simulink model "COPIA03052018"  (R2016a)
settings: Solver=ode3  StartTime=0.0  StopTime=inf  FixedStep=h  RelTol=1e-3
undefined symbols (not defined in the file): h, National_Instruments, PCI
libraries: sldrtlib x4, fuzblock x1
settings Model: SimulationMode=external  Creator=Jovani  LastModifiedBy=MCAC-UAEH
settings DataIOCC: LimitDataPoints=on  SaveFormat=Array
settings DebuggingCC: UnderspecifiedInitializationDetection=Classic  MergeDetectMultiDrivingBlocksExec=none  SolverPrmCheckMsg=warning  StateNameClashWarn=warning
settings HardwareCC: ProdBitPerLong=64  ProdLargestAtomicFloat=None  ProdHWDeviceType=Intel->x86-64  TargetBitPerLong=64  TargetBitPerPointer=64  TargetIntDivRoundTo=Zero  TargetEndianess=LittleEndian  TargetWordSize=64  TargetHWDeviceType=Intel->x86-64
settings ModelReferenceCC: PropagateSignalLabelsOutOfModel=off
settings RTWCC: SystemTargetFile=sldrt.tlc  TemplateMakefile=sldrt.tmf  Description=Simulink Desktop Real-Time  RTWCompilerOptimization=on
settings CodeAppCC: MaxIdLength=95
settings SimulinkDesktopRealTimeCC: TargetPreCompLibLocation=C:\Program Files\MATLAB\R2016a\toolbox\sldrt\lib\win64  TargetLangStandard=C89/C90 (ANSI)  SupportVariableSizeSignals=off
settings ConfigComp: CovModelRefEnable=Off

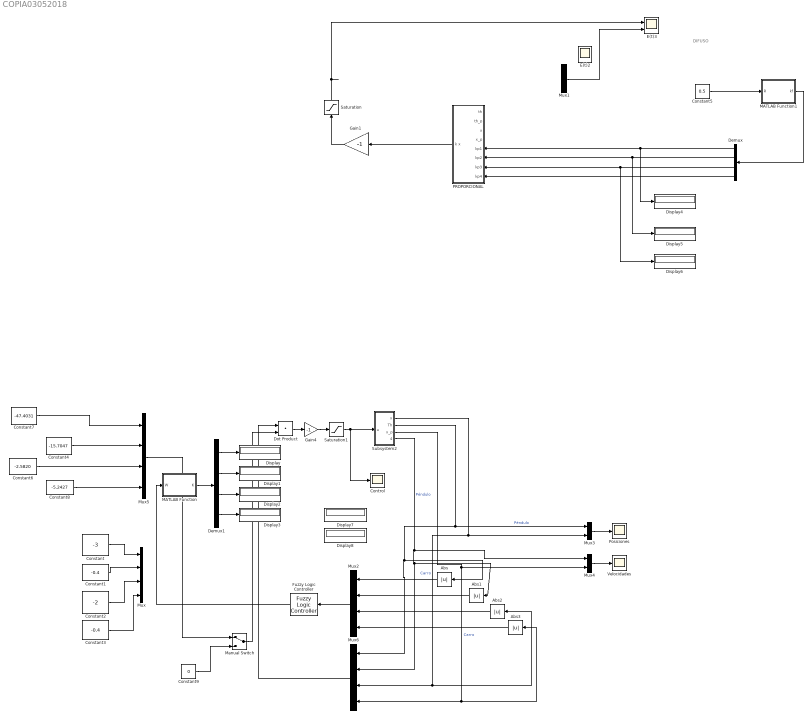
== system COPIA03052018 ==
  note: DIFUSO
  Abs{,1..3} (4 alike) : Abs
  Constant : Constant  Value=-3
  Constant1 : Constant  Value=-0.4
  Constant2 : Constant  Value=-2
  Constant3 : Constant  Value=-0.4
  Constant4 : Constant  Value=-15.7047
  Constant5 : Constant  Value=0.5
  Constant6 : Constant  Value=-2.5820
  Constant7 : Constant  Value=-47.4031
  Constant8 : Constant  Value=-5.2427
  Constant9 : Constant  Value=0
  "Control " : Scope
  Demux : Demux
  Demux1 : Demux
  Display{,1..8} (9 alike) : Display
  Dot Product : DotProduct  InputSameDT=on  OutDataTypeStr=Inherit: Inherit via internal rule
  E(t)2 : Scope  NumInputPorts=4
  E(t)3 : Scope  NumInputPorts=2
  Fuzzy Logic Controller : fuzblock/Fuzzy Logic  Controller  fis=P_T
  Gain1 : Gain  Gain=-1
  Gain4 : Gain  Gain=-1
  MATLAB Function : MATLAB Function  TreatAsAtomicUnit=on
  MATLAB Function1 : MATLAB Function  TreatAsAtomicUnit=on
  Manual Switch : ManualSwitch
  Mux{,1..2,5..6} (5 alike) : Mux
  Mux3 : Mux  Inputs=2
  Mux4 : Mux  Inputs=2
  PROPORCIONAL : Subsystem
  Posiciones : Scope
  Saturation : Saturate  UpperLimit=7.5  LowerLimit=-7.5
  Saturation1 : Saturate  UpperLimit=7.5  LowerLimit=-7.5
  Subsystem2 : Subsystem
  Velocidades : Scope
  wires:
  Gain1/1 -> Saturation/1
  ? -> PROPORCIONAL/2(th_p), Mux1/4, E(t)2/3
  ? -> E(t)2/4, Mux1/3, PROPORCIONAL/4(x_p)
  ? -> E(t)2/2, Mux1/2, PROPORCIONAL/1(th)
  ? -> E(t)2/1, Mux1/1, PROPORCIONAL/3(x)
  Mux1/1 -> E(t)3/2
  PROPORCIONAL/1(k x) -> Gain1/1
  Saturation/1 -> E(t)3/1
  Constant5/1 -> MATLAB Function1/1(R)
  MATLAB Function1/1(kf) -> Demux/1
  Demux/1 -> Display4/1, PROPORCIONAL/5(kp1)
  Demux/2 -> Display5/1, PROPORCIONAL/6(kp2)
  Demux/3 -> Display6/1, PROPORCIONAL/7(kp3)
  Demux/4 -> PROPORCIONAL/8(kp4)
  Demux1/1 -> Display/1
  Demux1/2 -> Display1/1
  Demux1/3 -> Display2/1
  Demux1/4 -> Display3/1
  MATLAB Function/1(K) -> Demux1/1
  Dot Product/1 -> Gain4/1
  Mux3/1 -> Posiciones/1
  Mux4/1 -> Velocidades/1
  Subsystem2/1(x) -> Mux3/2, Mux6/3, Abs2/1  "Carro"
  Subsystem2/4(th_p) -> Mux6/2, Abs1/1, Mux4/1  "Péndulo"
  Subsystem2/2(Th) -> Mux3/1, Mux6/1, Abs/1  "Péndulo"
  Subsystem2/3(x_p) -> Mux6/4, Abs3/1, Mux4/2  "Carro"
  Abs/1 -> Mux2/1
  Abs1/1 -> Mux2/2
  Abs2/1 -> Mux2/3
  Abs3/1 -> Mux2/4
  Constant/1 -> Mux/1
  Constant1/1 -> Mux/2
  Constant2/1 -> Mux/3
  Constant3/1 -> Mux/4
  Constant6/1 -> Mux5/3
  Constant7/1 -> Mux5/1
  Constant4/1 -> Mux5/2
  Constant8/1 -> Mux5/4
  Mux5/1 -> Manual Switch/1
  Constant9/1 -> Manual Switch/2
  Manual Switch/1 -> Dot Product/2
  Mux6/1 -> Dot Product/1
  Mux2/1 -> Fuzzy Logic Controller/1
  Fuzzy Logic Controller/1 -> MATLAB Function/1(W)
  Gain4/1 -> Saturation1/1
  Saturation1/1 -> "Control "/1, Subsystem2/1(u)

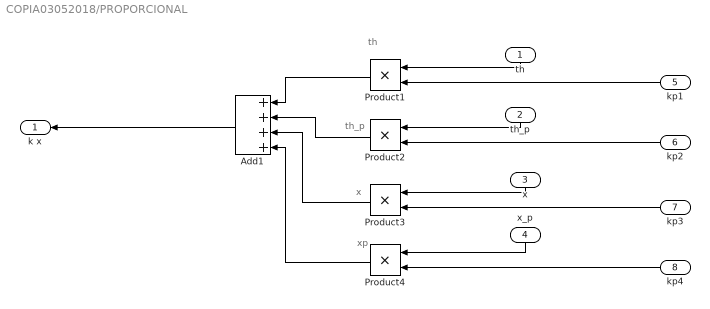
== system COPIA03052018/PROPORCIONAL ==
  note: xp
  note: x
  note: th_p
  note: th
  th : Inport
  th_p : Inport  Port=2
  x : Inport  Port=3
  x_p : Inport  Port=4
  kp1 : Inport  Port=5
  kp2 : Inport  Port=6
  kp3 : Inport  Port=7
  kp4 : Inport  Port=8
  Add1 : Sum  Inputs=++++
  Product{1..4} (4 alike) : Product
  k x : Outport
  wires:
  x_p/1 -> Product4/1
  x/1 -> Product3/1
  th_p/1 -> Product2/1
  th/1 -> Product1/1
  Add1/1 -> k x/1
  Product4/1 -> Add1/4
  Product3/1 -> Add1/3
  Product2/1 -> Add1/2
  Product1/1 -> Add1/1
  kp3/1 -> Product3/2
  kp1/1 -> Product1/2
  kp2/1 -> Product2/2
  kp4/1 -> Product4/2

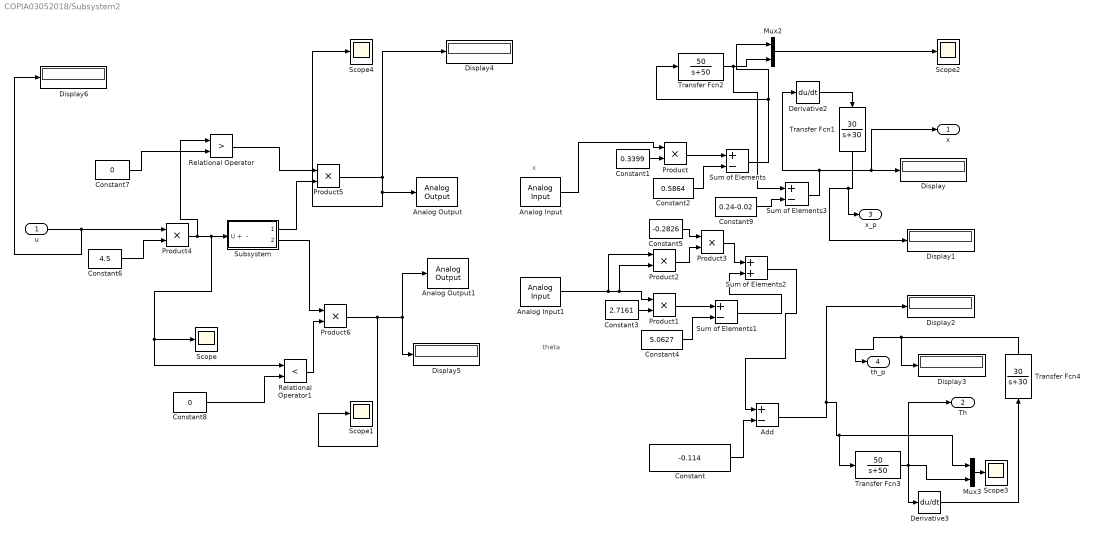
== system COPIA03052018/Subsystem2 ==
  note: x
  note: theta
  u : Inport
  Add : Sum  Inputs=+-
  Analog Input : sldrtlib/Analog Input  SampleTime=h  MaxMissedTicks=10  ShowMissedTicks=off  YieldWhenWaiting=off  DrvName=National_Instruments/PCI-6071E  DrvAddress=0  DrvOptions=[0 0 0 0 0 0]  Channels=1  RangeMode=1  VoltRange=10  DataType=1
      settings: AttributesFormatString=National Instruments\nPCI-6071E [0h]
  Analog Input1 : sldrtlib/Analog Input  SampleTime=h  MaxMissedTicks=10  ShowMissedTicks=off  YieldWhenWaiting=off  DrvName=National_Instruments/PCI-6071E  DrvAddress=0  DrvOptions=[0 0 0 0 0 0]  Channels=2  RangeMode=1  VoltRange=10  DataType=1
      settings: AttributesFormatString=National Instruments\nPCI-6071E [0h]
  Analog Output : sldrtlib/Analog Output  SampleTime=h  MaxMissedTicks=10  ShowMissedTicks=off  YieldWhenWaiting=off  DrvName=National_Instruments/PCI-6071E  DrvAddress=0  DrvOptions=[0 0 0 0 0 0]  Channels=1  RangeMode=1  VoltRange=1  InitialValue=[]  FinalValue=[]
      settings: AttributesFormatString=National Instruments\nPCI-6071E [0h]
  Analog Output1 : sldrtlib/Analog Output  SampleTime=h  MaxMissedTicks=10  ShowMissedTicks=off  YieldWhenWaiting=off  DrvName=National_Instruments/PCI-6071E  DrvAddress=0  DrvOptions=[0 0 0 0 0 0]  Channels=2  RangeMode=1  VoltRange=1  InitialValue=[]  FinalValue=[]
      settings: AttributesFormatString=National Instruments\nPCI-6071E [0h]
  Constant : Constant  Value=-0.114
  Constant1 : Constant  Value=0.3399
  Constant2 : Constant  Value=0.5864
  Constant3 : Constant  Value=2.7161
  Constant4 : Constant  Value=5.0627
  Constant5 : Constant  Value=-0.2826
  Constant6 : Constant  Value=4.5
  Constant7 : Constant  Value=0
  Constant8 : Constant  Value=0
  Constant9 : Constant  Value=0.24-0.02
  Derivative2 : Derivative
  Derivative3 : Derivative
  Display{,1..6} (7 alike) : Display
  Mux2 : Mux  Inputs=2
  Mux3 : Mux  Inputs=2
  Product{,1..6} (7 alike) : Product
  Relational Operator : RelationalOperator  Operator=>  OutDataTypeStr=boolean
  Relational Operator1 : RelationalOperator  Operator=<  OutDataTypeStr=boolean
  Scope{,1..4} (5 alike) : Scope
  Subsystem : Subsystem
  Sum of Elements : Sum  Inputs=+-
  Sum of Elements1 : Sum  Inputs=+-
  Sum of Elements2 : Sum
  Sum of Elements3 : Sum  Inputs=+-
  Transfer Fcn1 : TransferFcn  Numerator=[30]  Denominator=[1 30]
  Transfer Fcn2 : TransferFcn  Numerator=[50]  Denominator=[1 50]
  Transfer Fcn3 : TransferFcn  Numerator=[50]  Denominator=[1 50]
  Transfer Fcn4 : TransferFcn  Numerator=[30]  Denominator=[1 30]
  x : Outport
  Th : Outport  Port=2
  x_p : Outport  Port=3
  th_p : Outport  Port=4
  wires:
  Transfer Fcn4/1 -> th_p/1, Display3/1
  Transfer Fcn1/1 -> x_p/1, Display1/1
  Transfer Fcn3/1 -> Mux3/2, Derivative3/1, Th/1
  Mux3/1 -> Scope3/1
  Transfer Fcn2/1 -> Mux2/2, Sum of Elements3/1
  Mux2/1 -> Scope2/1
  Derivative3/1 -> Transfer Fcn4/1
  Derivative2/1 -> Transfer Fcn1/1
  Subsystem/2(neg ++) -> Product6/1
  Subsystem/1(pos ++) -> Product5/2
  Constant/1 -> Add/2
  Sum of Elements2/1 -> Add/1
  Relational Operator/1 -> Product5/1
  Product6/1 -> Scope1/1, Analog Output1/1, Display5/1
  Relational Operator1/1 -> Product6/2
  Constant8/1 -> Relational Operator1/2
  Product5/1 -> Scope4/1, Analog Output/1, Display4/1
  Constant7/1 -> Relational Operator/2
  Product4/1 -> Subsystem/1(U +  -), Scope/1, Relational Operator1/1, Relational Operator/1
  Constant6/1 -> Product4/2
  u/1 -> Product4/1, Display6/1
  Sum of Elements1/1 -> Sum of Elements2/2
  Product3/1 -> Sum of Elements2/1
  Product2/1 -> Product3/2
  Constant5/1 -> Product3/1
  Constant4/1 -> Sum of Elements1/2
  Constant3/1 -> Product1/2
  Product1/1 -> Sum of Elements1/1
  Sum of Elements/1 -> Transfer Fcn2/1, Mux2/1
  Constant2/1 -> Sum of Elements/2
  Constant1/1 -> Product/2
  Product/1 -> Sum of Elements/1
  Analog Input/1 -> Product/1
  Analog Input1/1 -> Product1/1, Product2/2, Product2/1
  Add/1 -> Mux3/1, Transfer Fcn3/1, Display2/1
  Constant9/1 -> Sum of Elements3/2
  Sum of Elements3/1 -> x/1, Display/1, Derivative2/1

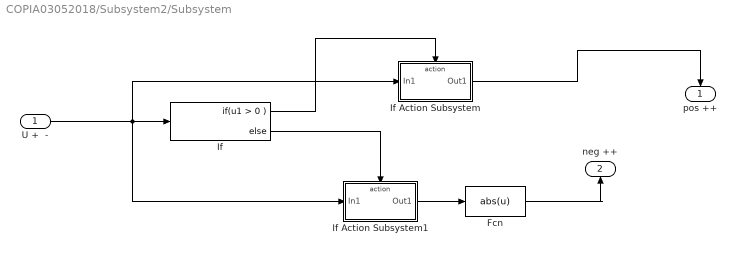
== system COPIA03052018/Subsystem2/Subsystem ==
  U +  - : Inport
  Fcn : Fcn  Expr=abs(u)
  If : If  IfExpression=u1 > 0
  If Action Subsystem : Subsystem  TreatAsAtomicUnit=on
  If Action Subsystem1 : Subsystem  TreatAsAtomicUnit=on
  pos ++ : Outport
  neg ++ : Outport  Port=2
  wires:
  Fcn/1 -> neg ++/1
  If Action Subsystem1/1(Out1) -> Fcn/1
  If Action Subsystem/1(Out1) -> pos ++/1
  If/2 -> If Action Subsystem1/Action
  U +  -/1 -> If/1, If Action Subsystem/1(In1), If Action Subsystem1/1(In1)
  If/1 -> If Action Subsystem/Action

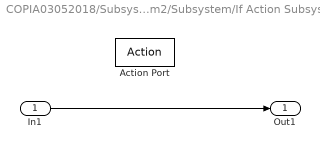
== system COPIA03052018/Subsystem2/Subsystem/If Action Subsystem ==
  In1 : Inport
  Action Port : ActionPort  ActionType=then
  Out1 : Outport
  wires:
  In1/1 -> Out1/1

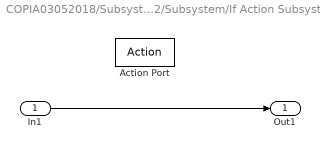
== system COPIA03052018/Subsystem2/Subsystem/If Action Subsystem1 ==
  In1 : Inport
  Action Port : ActionPort  ActionType=else
  Out1 : Outport
  wires:
  In1/1 -> Out1/1

== matlab function COPIA03052018/MATLAB Function1 ==
  data: R input; kf output
function kf = fcn(R)
%#codegen
%kf=[-60.1155,-15.6512,-6.3246,-10.4452];
kf=[-60.1155,-15.6512,-6.3246,-10.4452];

end

== matlab function COPIA03052018/MATLAB Function ==
  data: W input; K output
function K = fcn(W)
Wn1=W(1);
Xi1=W(2);
Wn2=W(3);
Xi2=W(4);
K3=Wn2^2*Wn1^2*(1/-7.3923);
K4=(1/-7.3923)*(2*Xi1*Wn1*Wn2^2+2*Xi2*Wn2*Wn1^2);
K1=(1/-0.755)*(Wn2^2+4*Xi1*Wn1*Xi2*Wn2+Wn1^2-5.92);
K2=(1/-0.755)*(2*Xi2*Wn2+2*Xi1*Wn1-0.6173*K4);

K=[K1 K2 K3 K4];
